simulink model "sm_abbYuMi_trajectory"  (R2021a)
settings: Solver=daessc  StartTime=0.0  StopTime=size(waypointsL, 2) * segment_duration  MaxStep=0.5  RelTol=1e-3  AbsTol=1e-3
values from neighbouring files (symbols this model uses):
  cube_l = 0.02    [startup_sm_abbYuMi_trajectory.m]
  segment_duration = 1.5    [sm_abbYuMi_trajectory_waypoints.m]    (also in startup_sm_abbYuMi_trajectory.m = 2)
undefined symbols (not defined in the file or in its folder): F1, F2, X, Y, Z
libraries: sm_lib x228, nesl_utility x52, robotcorelib x2
(part 1 of 6)
CloseFcn:
  | try,close(h1_sm_abbYuMi_trajectory),end
  | clear h1_sm_abbYuMi_2_trajectory
  | try,close(h2_sm_abbYuMi_trajectory),end
  | clear h2_sm_abbYuMi_2_trajectory
  | try,close(h3_sm_abbYuMi_trajectory),end
  | clear h3_sm_abbYuMi_2_trajectory
  | try,close(h4_sm_abbYuMi_trajectory),end
  | clear h4_sm_abbYuMi_trajectory
  | 
  | 
  | clear simlog_sm_abbYuMi_trajectory
  | clear logsout_sm_abbYuMi_trajectory
Description:
  | Dual Arm Robot Trajectory Testing
settings Model: Creator=smiller  LastModifiedBy=USER
settings SolverCC: AutoScaleAbsTol=off
settings DataIOCC: MaxDataPoints=10000  ReturnWorkspaceOutputs=off  SignalLoggingName=logsout_sm_abbYuMi_trajectory
settings SimscapeCC: SimscapeLogType=all  SimscapeLogSimulationStatistics=on  SimscapeLogName=simlog_sm_abbYuMi_trajectory  SimscapeLogDataHistory=10000
settings ExplorerConfigSet: InternalSimMechanicsExplorerSettings="<ExplorerConfiguration><canonicalview>default</canonicalview><AnimationSetting><BasePlaybackSpeed>1.0</BasePlaybackSpeed><PlaybackSpeedFactor>1.0</PlaybackSpeedFactor></AnimationSetting><TilePanel><TileInfo><Tiles Columns=\"1\" Count=\"1\" Rows=\"1\"><Column Weight=\"1\"/><Row Weight=\"1\"/><Tile Height=\"1\" Width=\"1\" X=\"0\" Y=\"0\"/></Tiles></TileInfo><SceneInfo><SceneViewer><BGColor><R>1</R><G>1</G><B>1</B></BGColor><Camera><DoPerspective>off</DoPerspective><Position><X>0.471611663595321084</X><Y>-0.677761083071622084</Y><Z>0.849724510093532892</Z></Position><Center><X>-0.196535950699227191</X><Y>-0.00961346877707375258</Y><Z>0.181576895798984672</Z></Center><Up><X>-0.408248290463863073</X><Y>0.408248290463863073</Y><Z>0.816496580927726145</Z></Up><ViewLimDist>1</ViewLimDist><YLim>0.557252171635627791</YLim><XLim>0.800218953628602181</XLim></Camera></SceneViewer></SceneInfo></TilePanel><MechEditorPanel><Cameras/><GfxPanelCameraMap/><VideoCreator><PlaybackSpeedRatio>1</PlaybackSpeedRatio><FrameRate>30</FrameRate><VideoFormat>MPEG-4</VideoFormat><FrameSize>auto</FrameSize></VideoCreator></MechEditorPanel></ExplorerConfiguration>"

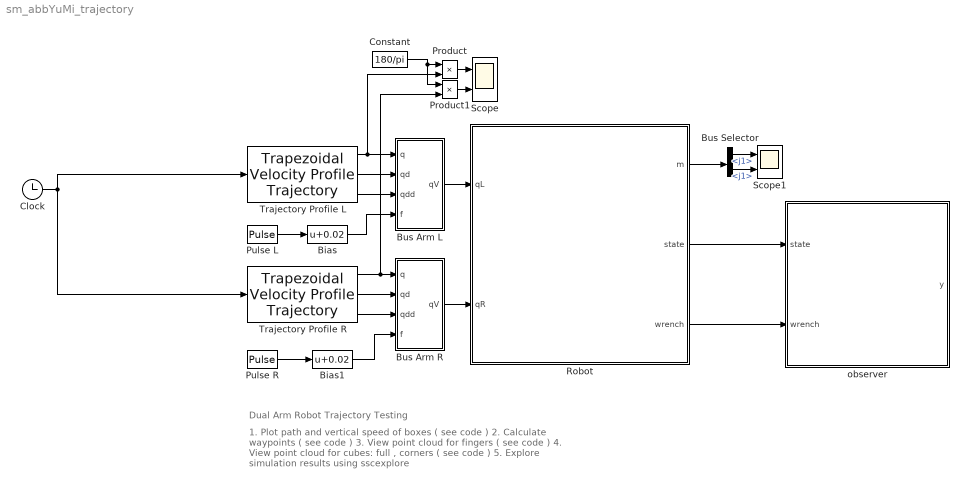
== system sm_abbYuMi_trajectory ==
  note: Dual Arm Robot Trajectory Testing
  note: 1. Plot path and vertical speed of boxes ( see code )
      | 2. Calculate waypoints ( see code )
      | 3. View point cloud for fingers ( see code )
      | 4. View point cloud for cubes: full , corners ( see code )
      | 5. Explore simulation results using sscexplore
  Bias : Bias  Bias=0.02
  Bias1 : Bias  Bias=0.02
  Bus Selector : BusSelector  OutputSignals=trqL.j1,trqR.j1
  Bus Arm L : Subsystem
  Bus Arm R : Subsystem
  Clock : Clock
  Constant : Constant  Value=180/pi
  Product : Product
  Product1 : Product
  Pulse L : DiscretePulseGenerator  PulseType=Time based  Amplitude=-0.011  Period=100  PulseWidth=4*segment_duration  PhaseDelay=2*segment_duration
  Pulse R : DiscretePulseGenerator  PulseType=Time based  Amplitude=-0.011  Period=100  PulseWidth=4*segment_duration  PhaseDelay=6*segment_duration
  Robot : Subsystem  mask(Dual Arm Robot with Contact Forces){k_gripBox=1e3, k_boxBox=1e3, k_boxFloor=1e3, d_gripBox=1e2, d_boxBox=1e2, d_boxFloor=1e2, t_gripBox=1e-3, t_boxBox=1e-3, t_boxFloor=1e-3, mu_s_gripBox=0.7, mu_s_boxBox=0.5, mu_s_boxFloor=0.5, mu_d_gripBox=0.5, mu_d_boxBox=0.3, mu_d_boxFloor=0.3, mu_v_gripBox=1e-3, mu_v_boxBox=1e-3, mu_v_boxFloor=1e-3}
      mask help: Models a dual-arm robot. Parameter values define the contact and friction forces between the gripper, boxes, and floor.
      mask DialogControl Control2_copy_copy_copy_copy_copy_copy_copy Prompt: Gripper-Box
      mask DialogControl Control2_copy_copy_copy_copy_copy_copy_copy_copy Prompt: Box-Box
      mask DialogControl Control2_copy_copy_copy_copy_copy_copy_copy_copy_copy Prompt: Box-Floor
      mask DialogControl Control2_copy_copy_copy_copy_copy_copy Prompt: Damping (N/(m/s))
      mask DialogControl Control2_copy Prompt: Damping (N/(m/s))
      mask DialogControl Control2_copy_copy Prompt: Transition Width (m)
      mask DialogControl Control2_copy_copy_copy Prompt: Static Friction (0-1)
      mask DialogControl Control2_copy_copy_copy_copy Prompt: Dynamic Friction (0-1)
      mask DialogControl Control2_copy_copy_copy_copy_copy Prompt: Critical Velocity (m/s)
      mask Display: image('sm_abbYuMi_trajectory_robot.png');
  Scope : Scope  NumInputPorts=2
  Scope1 : Scope  NumInputPorts=2
  Trajectory Profile L : robotcorelib/Trapezoidal Velocity Profile Trajectory  WaypointSource=Internal  Waypoints=waypointsL  NumParams=1  Parameter1=End Time  Parameter2=End Time  ParameterSource=Internal  PeakVelocity=[ 2; 2 ]  Acceleration=[ 1; 2 ]  EndTime=segment_duration  AccelTime=[ 1; 2 ]  SimulateUsing=Code generation
      settings: SourceProductBaseCode=NV,RO,RR,UV
  Trajectory Profile R : robotcorelib/Trapezoidal Velocity Profile Trajectory  WaypointSource=Internal  Waypoints=waypointsR  NumParams=1  Parameter1=End Time  Parameter2=End Time  ParameterSource=Internal  PeakVelocity=[ 2; 2 ]  Acceleration=[ 1; 2 ]  EndTime=segment_duration  AccelTime=[ 1; 2 ]  SimulateUsing=Code generation
      settings: SourceProductBaseCode=NV,RO,RR,UV
  observer : Subsystem
  wires:
  Clock/1 -> Trajectory Profile L/1, Trajectory Profile R/1
  Trajectory Profile L/1 -> Product/2, Bus Arm L/1(q)
  Trajectory Profile L/2 -> Bus Arm L/2(qd)
  Trajectory Profile L/3 -> Bus Arm L/3(qdd)
  Product/1 -> Scope/1
  Pulse L/1 -> Bias/1
  Trajectory Profile R/3 -> Bus Arm R/3(qdd)
  Trajectory Profile R/2 -> Bus Arm R/2(qd)
  Trajectory Profile R/1 -> Product1/2, Bus Arm R/1(q)
  Product1/1 -> Scope/2
  Pulse R/1 -> Bias1/1
  Bus Arm L/1(qV) -> Robot/1(qL)
  Constant/1 -> Product1/1, Product/1
  Bias1/1 -> Bus Arm R/4(f)
  Bias/1 -> Bus Arm L/4(f)
  Robot/1(m) -> Bus Selector/1
  Bus Selector/1 -> Scope1/1  "<j1>"
  Bus Selector/2 -> Scope1/2  "<j1>"
  Robot/2(state) -> observer/1(state)
  Robot/3(wrench) -> observer/2(wrench)
  Bus Arm R/1(qV) -> Robot/2(qR)

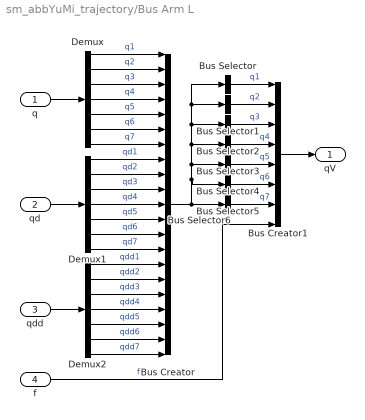
== system sm_abbYuMi_trajectory/Bus Arm L ==
  q : Inport
  qd : Inport  Port=2
  qdd : Inport  Port=3
  f : Inport  Port=4
  Bus Creator : BusCreator  Inputs=21
  Bus Creator1 : BusCreator  Inputs=8
  Bus Selector : BusSelector  OutputSignals=q1,qd1,qdd1  OutputAsBus=on
  Bus Selector1 : BusSelector  OutputSignals=q2,qd2,qdd2  OutputAsBus=on
  Bus Selector2 : BusSelector  OutputSignals=q3,qd3,qdd3  OutputAsBus=on
  Bus Selector3 : BusSelector  OutputSignals=q4,qd4,qdd4  OutputAsBus=on
  Bus Selector4 : BusSelector  OutputSignals=q5,qd5,qdd5  OutputAsBus=on
  Bus Selector5 : BusSelector  OutputSignals=q6,qd6,qdd6  OutputAsBus=on
  Bus Selector6 : BusSelector  OutputSignals=q7,qd7,qdd7  OutputAsBus=on
  Demux : Demux  Outputs=7
  Demux1 : Demux  Outputs=7
  Demux2 : Demux  Outputs=7
  qV : Outport
  wires:
  f/1 -> Bus Creator1/8  "f"
  q/1 -> Demux/1
  qd/1 -> Demux1/1
  qdd/1 -> Demux2/1
  Demux/1 -> Bus Creator/1  "q1"
  Demux/2 -> Bus Creator/2  "q2"
  Demux/3 -> Bus Creator/3  "q3"
  Demux/4 -> Bus Creator/4  "q4"
  Demux/5 -> Bus Creator/5  "q5"
  Demux/6 -> Bus Creator/6  "q6"
  Demux/7 -> Bus Creator/7  "q7"
  Demux1/1 -> Bus Creator/8  "qd1"
  Demux1/2 -> Bus Creator/9  "qd2"
  Demux1/3 -> Bus Creator/10  "qd3"
  Demux1/4 -> Bus Creator/11  "qd4"
  Demux1/5 -> Bus Creator/12  "qd5"
  Demux1/6 -> Bus Creator/13  "qd6"
  Demux1/7 -> Bus Creator/14  "qd7"
  Demux2/1 -> Bus Creator/15  "qdd1"
  Demux2/2 -> Bus Creator/16  "qdd2"
  Demux2/3 -> Bus Creator/17  "qdd3"
  Demux2/4 -> Bus Creator/18  "qdd4"
  Demux2/5 -> Bus Creator/19  "qdd5"
  Demux2/6 -> Bus Creator/20  "qdd6"
  Demux2/7 -> Bus Creator/21  "qdd7"
  Bus Creator/1 -> Bus Selector5/1, Bus Selector4/1, Bus Selector3/1, Bus Selector2/1, Bus Selector/1, Bus Selector1/1, Bus Selector6/1
  Bus Selector/1 -> Bus Creator1/1  "q1"
  Bus Selector1/1 -> Bus Creator1/2  "q2"
  Bus Selector2/1 -> Bus Creator1/3  "q3"
  Bus Selector3/1 -> Bus Creator1/4  "q4"
  Bus Selector4/1 -> Bus Creator1/5  "q5"
  Bus Selector5/1 -> Bus Creator1/6  "q6"
  Bus Selector6/1 -> Bus Creator1/7  "q7"
  Bus Creator1/1 -> qV/1

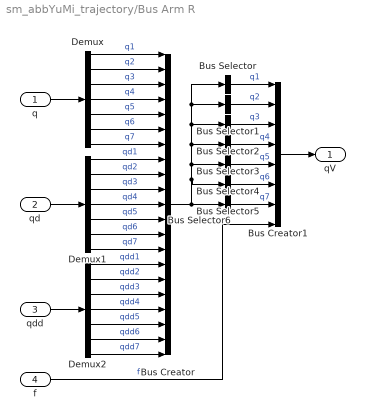
== system sm_abbYuMi_trajectory/Bus Arm R ==
  q : Inport
  qd : Inport  Port=2
  qdd : Inport  Port=3
  f : Inport  Port=4
  Bus Creator : BusCreator  Inputs=21
  Bus Creator1 : BusCreator  Inputs=8
  Bus Selector : BusSelector  OutputSignals=q1,qd1,qdd1  OutputAsBus=on
  Bus Selector1 : BusSelector  OutputSignals=q2,qd2,qdd2  OutputAsBus=on
  Bus Selector2 : BusSelector  OutputSignals=q3,qd3,qdd3  OutputAsBus=on
  Bus Selector3 : BusSelector  OutputSignals=q4,qd4,qdd4  OutputAsBus=on
  Bus Selector4 : BusSelector  OutputSignals=q5,qd5,qdd5  OutputAsBus=on
  Bus Selector5 : BusSelector  OutputSignals=q6,qd6,qdd6  OutputAsBus=on
  Bus Selector6 : BusSelector  OutputSignals=q7,qd7,qdd7  OutputAsBus=on
  Demux : Demux  Outputs=7
  Demux1 : Demux  Outputs=7
  Demux2 : Demux  Outputs=7
  qV : Outport
  wires:
  Bus Creator1/1 -> qV/1
  Bus Selector6/1 -> Bus Creator1/7  "q7"
  Bus Selector5/1 -> Bus Creator1/6  "q6"
  Bus Selector4/1 -> Bus Creator1/5  "q5"
  Bus Selector3/1 -> Bus Creator1/4  "q4"
  Bus Selector2/1 -> Bus Creator1/3  "q3"
  Bus Selector1/1 -> Bus Creator1/2  "q2"
  Bus Selector/1 -> Bus Creator1/1  "q1"
  Bus Creator/1 -> Bus Selector6/1, Bus Selector1/1, Bus Selector/1, Bus Selector2/1, Bus Selector3/1, Bus Selector4/1, Bus Selector5/1
  Demux2/7 -> Bus Creator/21  "qdd7"
  Demux2/6 -> Bus Creator/20  "qdd6"
  Demux2/5 -> Bus Creator/19  "qdd5"
  Demux2/4 -> Bus Creator/18  "qdd4"
  Demux2/3 -> Bus Creator/17  "qdd3"
  Demux2/2 -> Bus Creator/16  "qdd2"
  Demux2/1 -> Bus Creator/15  "qdd1"
  Demux1/7 -> Bus Creator/14  "qd7"
  Demux1/6 -> Bus Creator/13  "qd6"
  Demux1/5 -> Bus Creator/12  "qd5"
  Demux1/4 -> Bus Creator/11  "qd4"
  Demux1/3 -> Bus Creator/10  "qd3"
  Demux1/2 -> Bus Creator/9  "qd2"
  Demux1/1 -> Bus Creator/8  "qd1"
  Demux/7 -> Bus Creator/7  "q7"
  Demux/6 -> Bus Creator/6  "q6"
  Demux/5 -> Bus Creator/5  "q5"
  Demux/4 -> Bus Creator/4  "q4"
  Demux/3 -> Bus Creator/3  "q3"
  Demux/2 -> Bus Creator/2  "q2"
  Demux/1 -> Bus Creator/1  "q1"
  qdd/1 -> Demux2/1
  qd/1 -> Demux1/1
  q/1 -> Demux/1
  f/1 -> Bus Creator1/8  "f"

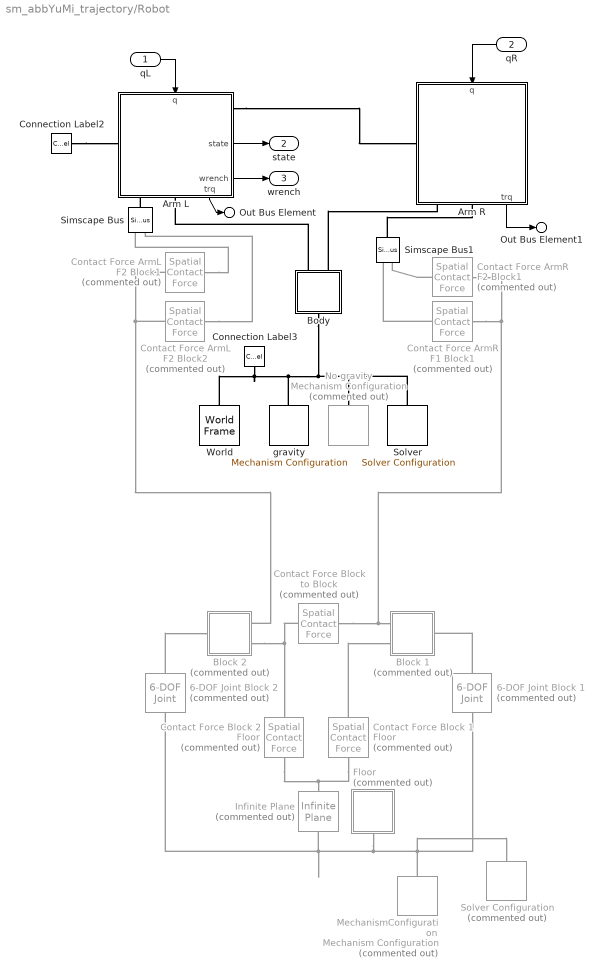
== system sm_abbYuMi_trajectory/Robot ==
  qL : Inport
  qR : Inport  Port=2
  " Contact Force Block to Block" : sm_lib/Forces and Torques/Spatial Contact Force  Commented=on  CoefficientOfDynamicFriction=mu_d_boxBox  CoefficientOfStaticFriction=mu_s_boxBox  SenseContactBaseRotation=off  SenseContactBaseTranslation=off  NormalDamping=d_boxBox  NormalDampingUnits=N/(m/s)  SenseContactFollowerRotation=off  SenseContactFollowerTranslation=off  SenseContactSignal=off  NormalStiffness=k_boxBox  NormalStiffnessUnits=N/m  FrictionalCriticalVelocity=mu_v_boxBox  FrictionalCriticalVelocityUnits=m/s  ZeroCrossDetectContactStartAndEnd=off  FrictionType=SmoothStickSlip  SenseFrictionalForceMagnitude=off  SenseNormalForceMagnitude=off  NormalForceType=SmoothSpringDamper  SenseNormalVelocity=off  SenseSeparationDistance=off  SenseTangentialVelocity=off  SenseTangentialVelocityMagnitude=off  NormalTransitionRegionWidth=t_boxBox  NormalTransitionRegionWidthUnits=m
  6-DOF Joint Block 1 : sm_lib/Joints/6-DOF Joint  Commented=on  JointMode=Normal  SenseConstraintForce=off  SenseConstraintForceX=off  SenseConstraintForceY=off  SenseConstraintForceZ=off  SenseConstraintTorque=off  SenseConstraintTorqueX=off  SenseConstraintTorqueY=off  SenseConstraintTorqueZ=off  SenseTotalForce=off  SenseTotalForceX=off  SenseTotalForceY=off  SenseTotalForceZ=off  SenseTotalTorque=off  SenseTotalTorqueX=off  SenseTotalTorqueY=off  SenseTotalTorqueZ=off  CompositeWrenchDir=FollowerOnBase  CompositeWrenchFrame=BaseFrame  PxEquilibriumPosition=0  PxEquilibriumPositionUnits=m  PxSpringStiffness=0  PxSpringStiffnessUnits=N/m  PxDampingCoefficient=0  PxDampingCoefficientUnits=N/(m/s)  PxTorqueActuationMode=NoTorque  PxMotionActuationMode=ComputedMotion  PxSensePosition=off  PxSenseVelocity=off  PxSenseAcceleration=off  PxSenseTorqueForce=off  PxSenseLowerLimitTorqueForce=off  PxSenseUpperLimitTorqueForce=off  PxLowerLimitSpecify=off  PxLowerLimitBound=-1  PxLowerLimitBoundUnits=m  PxLowerLimitStiffness=1e6  PxLowerLimitStiffnessUnits=N/m  PxLowerLimitDamping=1e3  PxLowerLimitDampingUnits=N/(m/s)  PxLowerLimitTransitionRegionWidth=1e-4  PxLowerLimitTransitionRegionWidthUnits=m  PxUpperLimitSpecify=off  PxUpperLimitBound=1  PxUpperLimitBoundUnits=m  PxUpperLimitStiffness=1e6  PxUpperLimitStiffnessUnits=N/m  PxUpperLimitDamping=1e3  PxUpperLimitDampingUnits=N/(m/s)  PxUpperLimitTransitionRegionWidth=1e-4  PxUpperLimitTransitionRegionWidthUnits=m  PxPositionTargetSpecify=on  PxPositionTargetPriority=High  PxPositionTargetValue=0.1  PxPositionTargetValueUnits=m  PxVelocityTargetSpecify=off  PxVelocityTargetPriority=High  PxVelocityTargetValue=0  PxVelocityTargetValueUnits=m/s  PyEquilibriumPosition=0  PyEquilibriumPositionUnits=m  PySpringStiffness=0  PySpringStiffnessUnits=N/m  PyDampingCoefficient=0  PyDampingCoefficientUnits=N/(m/s)  PyTorqueActuationMode=NoTorque  PyMotionActuationMode=ComputedMotion  PySensePosition=off  PySenseVelocity=off  PySenseAcceleration=off  PySenseTorqueForce=off  PySenseLowerLimitTorqueForce=off  PySenseUpperLimitTorqueForce=off  PyLowerLimitSpecify=off  PyLowerLimitBound=-1  PyLowerLimitBoundUnits=m  PyLowerLimitStiffness=1e6  PyLowerLimitStiffnessUnits=N/m  PyLowerLimitDamping=1e3  PyLowerLimitDampingUnits=N/(m/s)  PyLowerLimitTransitionRegionWidth=1e-4  PyLowerLimitTransitionRegionWidthUnits=m  PyUpperLimitSpecify=off  PyUpperLimitBound=1  PyUpperLimitBoundUnits=m  PyUpperLimitStiffness=1e6  PyUpperLimitStiffnessUnits=N/m  PyUpperLimitDamping=1e3  PyUpperLimitDampingUnits=N/(m/s)  PyUpperLimitTransitionRegionWidth=1e-4  PyUpperLimitTransitionRegionWidthUnits=m  PyPositionTargetSpecify=on  PyPositionTargetPriority=High  PyPositionTargetValue=-0.3  PyPositionTargetValueUnits=m  PyVelocityTargetSpecify=off  PyVelocityTargetPriority=High  PyVelocityTargetValue=0  PyVelocityTargetValueUnits=m/s  PzEquilibriumPosition=0  PzEquilibriumPositionUnits=m  PzSpringStiffness=0  PzSpringStiffnessUnits=N/m  PzDampingCoefficient=0  PzDampingCoefficientUnits=N/(m/s)  PzTorqueActuationMode=NoTorque  PzMotionActuationMode=ComputedMotion  PzSensePosition=off  PzSenseVelocity=off  PzSenseAcceleration=off  PzSenseTorqueForce=off  PzSenseLowerLimitTorqueForce=off  PzSenseUpperLimitTorqueForce=off  PzLowerLimitSpecify=off  PzLowerLimitBound=0  PzLowerLimitBoundUnits=m  PzLowerLimitStiffness=1e6  PzLowerLimitStiffnessUnits=N/m  PzLowerLimitDamping=1e3  PzLowerLimitDampingUnits=N/(m/s)  PzLowerLimitTransitionRegionWidth=1e-4  PzLowerLimitTransitionRegionWidthUnits=m  PzUpperLimitSpecify=off  PzUpperLimitBound=1  PzUpperLimitBoundUnits=m  PzUpperLimitStiffness=1e6  PzUpperLimitStiffnessUnits=N/m  PzUpperLimitDamping=1e3  PzUpperLimitDampingUnits=N/(m/s)  PzUpperLimitTransitionRegionWidth=1e-4  PzUpperLimitTransitionRegionWidthUnits=m  PzPositionTargetSpecify=on  PzPositionTargetPriority=High  PzPositionTargetValue=0.011  PzPositionTargetValueUnits=m  PzVelocityTargetSpecify=off  PzVelocityTargetPriority=High  PzVelocityTargetValue=0  PzVelocityTargetValueUnits=m/s  SphDefPosRotationMethod=None  SphDefPosRotationAngleUnits=deg  SphDefPosRotationStandardAxis=+Z  SphDefPosRotationAngle=0.0  SphDefPosRotationArbitraryAxis=[0 0 1]  SphDefPosFollAlignAxisA=+X  SphDefPosBaseAlignAxisA=+Y  SphDefPosFollAlignAxisB=+Y  SphDefPosBaseAlignAxisB=+Z  SphDefPosRotationSequenceAxes=FollowerAxes  SphDefPosRotationSequence=XYX  SphDefPosRotationSequenceAngles=[0 0 0]  SphDefPosRotationSequenceAnglesUnits=deg  SphDefPosRotationMatrix=[1 0 0; 0 1 0; 0 0 1]  SphEqPosRotationMethod=None  SphEqPosRotationAngleUnits=deg  SphEqPosRotationStandardAxis=+Z  SphEqPosRotationAngle=0.0  SphEqPosRotationArbitraryAxis=[0 0 1]  SphEqPosFollAlignAxisA=+X  SphEqPosBaseAlignAxisA=+Y  SphEqPosFollAlignAxisB=+Y  SphEqPosBaseAlignAxisB=+Z  SphEqPosRotationSequenceAxes=FollowerAxes  SphEqPosRotationSequence=XYX  SphEqPosRotationSequenceAngles=[0 0 0]  SphEqPosRotationSequenceAnglesUnits=deg  SphEqPosRotationMatrix=[1 0 0; 0 1 0; 0 0 1]  SphSpringStiffness=0  SphSpringStiffnessUnits=N*m/deg  SphDampingCoefficient=0  SphDampingCoefficientUnits=N*m/(deg/s)  SphActuateTorqueX=off  SphActuateTorqueY=off  SphActuateTorqueZ=off  SphActuateTorque=off  SphTorqueActuationMode=NoTorque  SphMotionActuationMode=ComputedMotion  SphActuationFrame=BaseFrame  SphSensePosition=off  SphSenseVelocityX=off  SphSenseVelocityY=off  SphSenseVelocityZ=off  SphSenseVelocity=off  SphSenseAccelerationX=off  SphSenseAccelerationY=off  SphSenseAccelerationZ=off  SphSenseAcceleration=off  SphSenseTorqueX=off  SphSenseTorqueY=off  SphSenseTorqueZ=off  SphSenseTorqueForce=off  SphSenseLowerLimitTorqueMag=off  SphSenseUpperLimitTorqueMag=off  SphSensingFrame=BaseFrame  SphLowerLimitSpecify=off  SphLowerLimitBound=15  SphLowerLimitBoundUnits=deg  SphLowerLimitStiffness=1e4  SphLowerLimitStiffnessUnits=N*m/deg  SphLowerLimitDamping=10  SphLowerLimitDampingUnits=N*m/(deg/s)  SphLowerLimitTransitionRegionWidth=0.1  SphLowerLimitTransitionRegionWidthUnits=deg  SphUpperLimitSpecify=off  SphUpperLimitBound=45  SphUpperLimitBoundUnits=deg  SphUpperLimitStiffness=1e4  SphUpperLimitStiffnessUnits=N*m/deg  SphUpperLimitDamping=10  SphUpperLimitDampingUnits=N*m/(deg/s)  SphUpperLimitTransitionRegionWidth=0.1  SphUpperLimitTransitionRegionWidthUnits=deg  SphPositionTargetRotationMethod=None  SphPositionTargetRotationAngleUnits=deg  SphPositionTargetRotationStandardAxis=+Z  SphPositionTargetRotationAngle=0.0  SphPositionTargetRotationArbitraryAxis=[0 0 1]  SphPositionTargetFollAlignAxisA=+X  SphPositionTargetBaseAlignAxisA=+Y  SphPositionTargetFollAlignAxisB=+Y  SphPositionTargetBaseAlignAxisB=+Z  SphPositionTargetRotationSequenceAxes=FollowerAxes  SphPositionTargetRotationSequence=XYX  SphPositionTargetRotationSequenceAngles=[0 0 0]  SphPositionTargetRotationSequenceAnglesUnits=deg  SphPositionTargetRotationMatrix=[1 0 0; 0 1 0; 0 0 1]  SphPositionTargetSpecify=off  SphPositionTargetPriority=High  SphVelocityTargetValue=[0 0 0]  SphVelocityTargetValueUnits=deg/s  SphVelocityTargetSpecify=off  SphVelocityTargetPriority=High  SphVelocityTargetInFollowerFrame=on
  6-DOF Joint Block 2 : sm_lib/Joints/6-DOF Joint  Commented=on  JointMode=Normal  SenseConstraintForce=off  SenseConstraintForceX=off  SenseConstraintForceY=off  SenseConstraintForceZ=off  SenseConstraintTorque=off  SenseConstraintTorqueX=off  SenseConstraintTorqueY=off  SenseConstraintTorqueZ=off  SenseTotalForce=off  SenseTotalForceX=off  SenseTotalForceY=off  SenseTotalForceZ=off  SenseTotalTorque=off  SenseTotalTorqueX=off  SenseTotalTorqueY=off  SenseTotalTorqueZ=off  CompositeWrenchDir=FollowerOnBase  CompositeWrenchFrame=BaseFrame  PxEquilibriumPosition=0  PxEquilibriumPositionUnits=m  PxSpringStiffness=0  PxSpringStiffnessUnits=N/m  PxDampingCoefficient=0  PxDampingCoefficientUnits=N/(m/s)  PxTorqueActuationMode=NoTorque  PxMotionActuationMode=ComputedMotion  PxSensePosition=off  PxSenseVelocity=off  PxSenseAcceleration=off  PxSenseTorqueForce=off  PxSenseLowerLimitTorqueForce=off  PxSenseUpperLimitTorqueForce=off  PxLowerLimitSpecify=off  PxLowerLimitBound=-1  PxLowerLimitBoundUnits=m  PxLowerLimitStiffness=1e6  PxLowerLimitStiffnessUnits=N/m  PxLowerLimitDamping=1e3  PxLowerLimitDampingUnits=N/(m/s)  PxLowerLimitTransitionRegionWidth=1e-4  PxLowerLimitTransitionRegionWidthUnits=m  PxUpperLimitSpecify=off  PxUpperLimitBound=1  PxUpperLimitBoundUnits=m  PxUpperLimitStiffness=1e6  PxUpperLimitStiffnessUnits=N/m  PxUpperLimitDamping=1e3  PxUpperLimitDampingUnits=N/(m/s)  PxUpperLimitTransitionRegionWidth=1e-4  PxUpperLimitTransitionRegionWidthUnits=m  PxPositionTargetSpecify=on  PxPositionTargetPriority=High  PxPositionTargetValue=0.1  PxPositionTargetValueUnits=m  PxVelocityTargetSpecify=off  PxVelocityTargetPriority=High  PxVelocityTargetValue=0  PxVelocityTargetValueUnits=m/s  PyEquilibriumPosition=0  PyEquilibriumPositionUnits=m  PySpringStiffness=0  PySpringStiffnessUnits=N/m  PyDampingCoefficient=0  PyDampingCoefficientUnits=N/(m/s)  PyTorqueActuationMode=NoTorque  PyMotionActuationMode=ComputedMotion  PySensePosition=off  PySenseVelocity=off  PySenseAcceleration=off  PySenseTorqueForce=off  PySenseLowerLimitTorqueForce=off  PySenseUpperLimitTorqueForce=off  PyLowerLimitSpecify=off  PyLowerLimitBound=-1  PyLowerLimitBoundUnits=m  PyLowerLimitStiffness=1e6  PyLowerLimitStiffnessUnits=N/m  PyLowerLimitDamping=1e3  PyLowerLimitDampingUnits=N/(m/s)  PyLowerLimitTransitionRegionWidth=1e-4  PyLowerLimitTransitionRegionWidthUnits=m  PyUpperLimitSpecify=off  PyUpperLimitBound=1  PyUpperLimitBoundUnits=m  PyUpperLimitStiffness=1e6  PyUpperLimitStiffnessUnits=N/m  PyUpperLimitDamping=1e3  PyUpperLimitDampingUnits=N/(m/s)  PyUpperLimitTransitionRegionWidth=1e-4  PyUpperLimitTransitionRegionWidthUnits=m  PyPositionTargetSpecify=on  PyPositionTargetPriority=High  PyPositionTargetValue=0.3  PyPositionTargetValueUnits=m  PyVelocityTargetSpecify=off  PyVelocityTargetPriority=High  PyVelocityTargetValue=0  PyVelocityTargetValueUnits=m/s  PzEquilibriumPosition=0  PzEquilibriumPositionUnits=m  PzSpringStiffness=0  PzSpringStiffnessUnits=N/m  PzDampingCoefficient=0  PzDampingCoefficientUnits=N/(m/s)  PzTorqueActuationMode=NoTorque  PzMotionActuationMode=ComputedMotion  PzSensePosition=off  PzSenseVelocity=off  PzSenseAcceleration=off  PzSenseTorqueForce=off  PzSenseLowerLimitTorqueForce=off  PzSenseUpperLimitTorqueForce=off  PzLowerLimitSpecify=off  PzLowerLimitBound=0  PzLowerLimitBoundUnits=m  PzLowerLimitStiffness=1e6  PzLowerLimitStiffnessUnits=N/m  PzLowerLimitDamping=1e3  PzLowerLimitDampingUnits=N/(m/s)  PzLowerLimitTransitionRegionWidth=1e-4  PzLowerLimitTransitionRegionWidthUnits=m  PzUpperLimitSpecify=off  PzUpperLimitBound=1  PzUpperLimitBoundUnits=m  PzUpperLimitStiffness=1e6  PzUpperLimitStiffnessUnits=N/m  PzUpperLimitDamping=1e3  PzUpperLimitDampingUnits=N/(m/s)  PzUpperLimitTransitionRegionWidth=1e-4  PzUpperLimitTransitionRegionWidthUnits=m  PzPositionTargetSpecify=on  PzPositionTargetPriority=High  PzPositionTargetValue=0.011  PzPositionTargetValueUnits=m  PzVelocityTargetSpecify=off  PzVelocityTargetPriority=High  PzVelocityTargetValue=0  PzVelocityTargetValueUnits=m/s  SphDefPosRotationMethod=None  SphDefPosRotationAngleUnits=deg  SphDefPosRotationStandardAxis=+Z  SphDefPosRotationAngle=0.0  SphDefPosRotationArbitraryAxis=[0 0 1]  SphDefPosFollAlignAxisA=+X  SphDefPosBaseAlignAxisA=+Y  SphDefPosFollAlignAxisB=+Y  SphDefPosBaseAlignAxisB=+Z  SphDefPosRotationSequenceAxes=FollowerAxes  SphDefPosRotationSequence=XYX  SphDefPosRotationSequenceAngles=[0 0 0]  SphDefPosRotationSequenceAnglesUnits=deg  SphDefPosRotationMatrix=[1 0 0; 0 1 0; 0 0 1]  SphEqPosRotationMethod=None  SphEqPosRotationAngleUnits=deg  SphEqPosRotationStandardAxis=+Z  SphEqPosRotationAngle=0.0  SphEqPosRotationArbitraryAxis=[0 0 1]  SphEqPosFollAlignAxisA=+X  SphEqPosBaseAlignAxisA=+Y  SphEqPosFollAlignAxisB=+Y  SphEqPosBaseAlignAxisB=+Z  SphEqPosRotationSequenceAxes=FollowerAxes  SphEqPosRotationSequence=XYX  SphEqPosRotationSequenceAngles=[0 0 0]  SphEqPosRotationSequenceAnglesUnits=deg  SphEqPosRotationMatrix=[1 0 0; 0 1 0; 0 0 1]  SphSpringStiffness=0  SphSpringStiffnessUnits=N*m/deg  SphDampingCoefficient=0  SphDampingCoefficientUnits=N*m/(deg/s)  SphActuateTorqueX=off  SphActuateTorqueY=off  SphActuateTorqueZ=off  SphActuateTorque=off  SphTorqueActuationMode=NoTorque  SphMotionActuationMode=ComputedMotion  SphActuationFrame=BaseFrame  SphSensePosition=off  SphSenseVelocityX=off  SphSenseVelocityY=off  SphSenseVelocityZ=off  SphSenseVelocity=off  SphSenseAccelerationX=off  SphSenseAccelerationY=off  SphSenseAccelerationZ=off  SphSenseAcceleration=off  SphSenseTorqueX=off  SphSenseTorqueY=off  SphSenseTorqueZ=off  SphSenseTorqueForce=off  SphSenseLowerLimitTorqueMag=off  SphSenseUpperLimitTorqueMag=off  SphSensingFrame=BaseFrame  SphLowerLimitSpecify=off  SphLowerLimitBound=15  SphLowerLimitBoundUnits=deg  SphLowerLimitStiffness=1e4  SphLowerLimitStiffnessUnits=N*m/deg  SphLowerLimitDamping=10  SphLowerLimitDampingUnits=N*m/(deg/s)  SphLowerLimitTransitionRegionWidth=0.1  SphLowerLimitTransitionRegionWidthUnits=deg  SphUpperLimitSpecify=off  SphUpperLimitBound=45  SphUpperLimitBoundUnits=deg  SphUpperLimitStiffness=1e4  SphUpperLimitStiffnessUnits=N*m/deg  SphUpperLimitDamping=10  SphUpperLimitDampingUnits=N*m/(deg/s)  SphUpperLimitTransitionRegionWidth=0.1  SphUpperLimitTransitionRegionWidthUnits=deg  SphPositionTargetRotationMethod=None  SphPositionTargetRotationAngleUnits=deg  SphPositionTargetRotationStandardAxis=+Z  SphPositionTargetRotationAngle=0.0  SphPositionTargetRotationArbitraryAxis=[0 0 1]  SphPositionTargetFollAlignAxisA=+X  SphPositionTargetBaseAlignAxisA=+Y  SphPositionTargetFollAlignAxisB=+Y  SphPositionTargetBaseAlignAxisB=+Z  SphPositionTargetRotationSequenceAxes=FollowerAxes  SphPositionTargetRotationSequence=XYX  SphPositionTargetRotationSequenceAngles=[0 0 0]  SphPositionTargetRotationSequenceAnglesUnits=deg  SphPositionTargetRotationMatrix=[1 0 0; 0 1 0; 0 0 1]  SphPositionTargetSpecify=off  SphPositionTargetPriority=High  SphVelocityTargetValue=[0 0 0]  SphVelocityTargetValueUnits=deg/s  SphVelocityTargetSpecify=off  SphVelocityTargetPriority=High  SphVelocityTargetInFollowerFrame=on
  Arm L : Subsystem
      settings: PortSchema="{\"entries\":[{\"content\":{\"sides\":[{\"content\":{\"connectorIds\":[\"In1\"]},\"type\":\"ConnectorPlacement.EquallySpacedRectSide\",\"uuid\":\"bd1dcecf-d297-44c9-a9a5-35bbd8af8960\"},{\"content\":{\"connectorIds\":[\"Out1\",\"RConn1\",\"RConn2\"],\"side\":\"RIGHT\"},\"type\":\"ConnectorPlacement.EquallySpacedRectSide\",\"uuid\":\"baf14d35-3a07-4b12-83f0-83ffbc31cdf5\"},{\"content\":{\"connectorIds\":[\"LConn1\",\"Out2\",\"Out3\"],\"side\":\"TOP\"},\"type\":\"ConnectorPlacement.EquallySpacedRectSide\",\"uuid\":\"824d8d51-c42e-4dae-9a8c-2ffaab279e02\"},{\"content\":{\"connectorIds\":[\"RConn3\"],\"side\":\"BOTTOM\"},\"type\":\"ConnectorPlacement.EquallySpacedRectSide\",\"uuid\":\"ad6f5a81-da03-4abe-8c16-f1c9b20f9016\"}]},\"type\":\"ConnectorPlacement.EquallySpacedConnector\",\"uuid\":\"fe86daed-a59d-484b-b331-148b99957df6\"}],\"packageUris\":[\"http://schema.mathworks.com/mf0/Connector/R2020b\"],\"version\":\"1.0\"}"
  Arm R : Subsystem
      settings: PortSchema="{\"entries\":[{\"content\":{\"sides\":[{\"content\":{\"connectorIds\":[\"In1\"]},\"type\":\"ConnectorPlacement.EquallySpacedRectSide\",\"uuid\":\"a5483abb-2b55-4c80-92c1-57afb39286c9\"},{\"content\":{\"connectorIds\":[\"Out1\",\"RConn1\",\"RConn2\"],\"side\":\"RIGHT\"},\"type\":\"ConnectorPlacement.EquallySpacedRectSide\",\"uuid\":\"70e7c0c0-7b67-4471-83d4-ebce2c38e118\"},{\"content\":{\"connectorIds\":[],\"side\":\"TOP\"},\"type\":\"ConnectorPlacement.EquallySpacedRectSide\",\"uuid\":\"5c3252dc-82b7-4f09-980f-704b78bb4b1e\"},{\"content\":{\"connectorIds\":[\"RConn3\"],\"side\":\"BOTTOM\"},\"type\":\"ConnectorPlacement.EquallySpacedRectSide\",\"uuid\":\"dc850cf4-a88e-4fa0-b309-256fbdf4b05e\"}]},\"type\":\"ConnectorPlacement.EquallySpacedConnector\",\"uuid\":\"ac9f6d8b-81cb-4b9f-aec0-3731a82563a6\"}],\"packageUris\":[\"http://schema.mathworks.com/mf0/Connector/R2020b\"],\"version\":\"1.0\"}"
  Block 1 : Subsystem  Commented=on
  Block 2 : Subsystem  Commented=on
  Body : Subsystem
  Connection Label2 : ConnectionLabel  Label=W
  Connection Label3 : ConnectionLabel  Label=W
  Contact Force Block 1 Floor : sm_lib/Forces and Torques/Spatial Contact Force  Commented=on  CoefficientOfDynamicFriction=mu_d_boxFloor  CoefficientOfStaticFriction=mu_s_boxFloor  SenseContactBaseRotation=off  SenseContactBaseTranslation=off  NormalDamping=d_boxFloor  NormalDampingUnits=N/(m/s)  SenseContactFollowerRotation=off  SenseContactFollowerTranslation=off  SenseContactSignal=off  NormalStiffness=k_boxFloor  NormalStiffnessUnits=N/m  FrictionalCriticalVelocity=mu_v_boxFloor  FrictionalCriticalVelocityUnits=m/s  ZeroCrossDetectContactStartAndEnd=off  FrictionType=SmoothStickSlip  SenseFrictionalForceMagnitude=off  SenseNormalForceMagnitude=off  NormalForceType=SmoothSpringDamper  SenseNormalVelocity=off  SenseSeparationDistance=off  SenseTangentialVelocity=off  SenseTangentialVelocityMagnitude=off  NormalTransitionRegionWidth=t_boxFloor  NormalTransitionRegionWidthUnits=m
  Contact Force Block 2 Floor : sm_lib/Forces and Torques/Spatial Contact Force  Commented=on  CoefficientOfDynamicFriction=mu_d_boxFloor  CoefficientOfStaticFriction=mu_s_boxFloor  SenseContactBaseRotation=off  SenseContactBaseTranslation=off  NormalDamping=d_boxFloor  NormalDampingUnits=N/(m/s)  SenseContactFollowerRotation=off  SenseContactFollowerTranslation=off  SenseContactSignal=off  NormalStiffness=k_boxFloor  NormalStiffnessUnits=N/m  FrictionalCriticalVelocity=mu_v_boxFloor  FrictionalCriticalVelocityUnits=m/s  ZeroCrossDetectContactStartAndEnd=off  FrictionType=SmoothStickSlip  SenseFrictionalForceMagnitude=off  SenseNormalForceMagnitude=off  NormalForceType=SmoothSpringDamper  SenseNormalVelocity=off  SenseSeparationDistance=off  SenseTangentialVelocity=off  SenseTangentialVelocityMagnitude=off  NormalTransitionRegionWidth=t_boxFloor  NormalTransitionRegionWidthUnits=m
  Contact Force ArmL F2 Block1 : sm_lib/Forces and Torques/Spatial Contact Force  Commented=on  CoefficientOfDynamicFriction=mu_d_gripBox  CoefficientOfStaticFriction=mu_s_gripBox  SenseContactBaseRotation=off  SenseContactBaseTranslation=off  NormalDamping=d_gripBox  NormalDampingUnits=N/(m/s)  SenseContactFollowerRotation=off  SenseContactFollowerTranslation=off  SenseContactSignal=off  NormalStiffness=k_gripBox  NormalStiffnessUnits=N/m  FrictionalCriticalVelocity=mu_v_gripBox  FrictionalCriticalVelocityUnits=m/s  ZeroCrossDetectContactStartAndEnd=off  FrictionType=SmoothStickSlip  SenseFrictionalForceMagnitude=off  SenseNormalForceMagnitude=off  NormalForceType=SmoothSpringDamper  SenseNormalVelocity=off  SenseSeparationDistance=off  SenseTangentialVelocity=off  SenseTangentialVelocityMagnitude=off  NormalTransitionRegionWidth=t_gripBox  NormalTransitionRegionWidthUnits=m
  Contact Force ArmL F2 Block2 : sm_lib/Forces and Torques/Spatial Contact Force  Commented=on  CoefficientOfDynamicFriction=mu_d_gripBox  CoefficientOfStaticFriction=mu_s_gripBox  SenseContactBaseRotation=off  SenseContactBaseTranslation=off  NormalDamping=d_gripBox  NormalDampingUnits=N/(m/s)  SenseContactFollowerRotation=off  SenseContactFollowerTranslation=off  SenseContactSignal=off  NormalStiffness=k_gripBox  NormalStiffnessUnits=N/m  FrictionalCriticalVelocity=mu_v_gripBox  FrictionalCriticalVelocityUnits=m/s  ZeroCrossDetectContactStartAndEnd=off  FrictionType=SmoothStickSlip  SenseFrictionalForceMagnitude=off  SenseNormalForceMagnitude=off  NormalForceType=SmoothSpringDamper  SenseNormalVelocity=off  SenseSeparationDistance=off  SenseTangentialVelocity=off  SenseTangentialVelocityMagnitude=off  NormalTransitionRegionWidth=t_gripBox  NormalTransitionRegionWidthUnits=m
  Contact Force ArmR F1 Block1 : sm_lib/Forces and Torques/Spatial Contact Force  Commented=on  CoefficientOfDynamicFriction=mu_d_gripBox  CoefficientOfStaticFriction=mu_s_gripBox  SenseContactBaseRotation=off  SenseContactBaseTranslation=off  NormalDamping=d_gripBox  NormalDampingUnits=N/(m/s)  SenseContactFollowerRotation=off  SenseContactFollowerTranslation=off  SenseContactSignal=off  NormalStiffness=k_gripBox  NormalStiffnessUnits=N/m  FrictionalCriticalVelocity=mu_v_gripBox  FrictionalCriticalVelocityUnits=m/s  ZeroCrossDetectContactStartAndEnd=off  FrictionType=SmoothStickSlip  SenseFrictionalForceMagnitude=off  SenseNormalForceMagnitude=off  NormalForceType=SmoothSpringDamper  SenseNormalVelocity=off  SenseSeparationDistance=off  SenseTangentialVelocity=off  SenseTangentialVelocityMagnitude=off  NormalTransitionRegionWidth=t_gripBox  NormalTransitionRegionWidthUnits=m
  Contact Force ArmR F2 Block1 : sm_lib/Forces and Torques/Spatial Contact Force  Commented=on  CoefficientOfDynamicFriction=mu_d_gripBox  CoefficientOfStaticFriction=mu_s_gripBox  SenseContactBaseRotation=off  SenseContactBaseTranslation=off  NormalDamping=d_gripBox  NormalDampingUnits=N/(m/s)  SenseContactFollowerRotation=off  SenseContactFollowerTranslation=off  SenseContactSignal=off  NormalStiffness=k_gripBox  NormalStiffnessUnits=N/m  FrictionalCriticalVelocity=mu_v_gripBox  FrictionalCriticalVelocityUnits=m/s  ZeroCrossDetectContactStartAndEnd=off  FrictionType=SmoothStickSlip  SenseFrictionalForceMagnitude=off  SenseNormalForceMagnitude=off  NormalForceType=SmoothSpringDamper  SenseNormalVelocity=off  SenseSeparationDistance=off  SenseTangentialVelocity=off  SenseTangentialVelocityMagnitude=off  NormalTransitionRegionWidth=t_gripBox  NormalTransitionRegionWidthUnits=m
  Floor : Subsystem  Commented=on
  Infinite Plane : sm_lib/Curves and Surfaces/Infinite Plane  Commented=on  GraphicType=Rectangle  GraphicPlaneWidth=1  GraphicPlaneWidthUnits=m  GraphicPlaneHeight=1  GraphicPlaneHeightUnits=m  GraphicVisPropType=SimpleVisualProperties  GraphicDiffuseColor=[0.5 0.5 0.5]  GraphicOpacity=0.25  GraphicSpecularColor=[0.5 0.5 0.5 1.0]  GraphicAmbientColor=[0.15 0.15 0.15 1.0]  GraphicEmissiveColor=[0.0 0.0 0.0 1.0]  GraphicShininess=75
  MechanismConfiguration : sm_lib/Utilities/Mechanism Configuration  Commented=on  UniformGravity=Constant  GravityVector=[0 0 0]  GravityVectorUnits=m/s^2  GravityUnits=m/s^2  LinearizationDelta=0.001  JointModeTransitionNonlinearIterations=2
  No gravity : sm_lib/Utilities/Mechanism Configuration  Commented=on  UniformGravity=Constant  GravityVector=[0 0 0]  GravityVectorUnits=m/s^2  GravityUnits=m/s^2  LinearizationDelta=0.001  JointModeTransitionNonlinearIterations=2
  Simscape Bus : SimscapeBus  HierarchyStrings=F1;F2
  Simscape Bus1 : SimscapeBus  HierarchyStrings=F1;F2
  Solver : nesl_utility/Solver Configuration  PhysicalDomain=network_engine_domain  SubClassName=solver  LeftPortType=input  RightPortType=generic  Tones=[]  Harmonics=[]  SimulateNoise=off  Profile=off  UseLocalSampling=off  EnableSwitchedLinearOptims=on  FrequencyDomain=off  UseCCode=off  RelTol=0.001  AbsTol=1e-06  MinStep=1e-09  ToWorkspace=off  RevertToSquareIcSolve=off  NumHomotopyIterations=100  PhasorMode=off  PhasorModeNumHarmonics=1  DoDC=off  ResidualTolerance=1e-09  UseLocalSolver=off  LocalSolverChoice=NE_BACKWARD_EULER_ADVANCER  LocalSolverSampleTime=0.001  DoFixedCost=off  MaxNonlinIter=3  MaxModeIter=2  ComputeImpulses=off  ImpulseIterations=2  LinearAlgebra=auto  EquationFormulation=NE_TIME_EF  DelaysMemoryBudget=1024  AutomaticFiltering=on  FilteringTimeConstant=0.001  PartitionStorageMethod=AS_NEEDED  PartitionMemoryBudget=1024  PartitionMethod=ROBUST
      settings: SourceProductBaseCode=PW,SS
  Solver Configuration : nesl_utility/Solver Configuration  Commented=on  PhysicalDomain=network_engine_domain  SubClassName=solver  LeftPortType=input  RightPortType=generic  Tones=[]  Harmonics=[]  SimulateNoise=off  Profile=off  UseLocalSampling=off  EnableSwitchedLinearOptims=on  FrequencyDomain=off  UseCCode=off  RelTol=0.001  AbsTol=1e-06  MinStep=1e-09  ToWorkspace=off  RevertToSquareIcSolve=off  NumHomotopyIterations=100  PhasorMode=off  PhasorModeNumHarmonics=1  DoDC=off  ResidualTolerance=1e-09  UseLocalSolver=off  LocalSolverChoice=NE_BACKWARD_EULER_ADVANCER  LocalSolverSampleTime=0.001  DoFixedCost=off  MaxNonlinIter=3  MaxModeIter=2  ComputeImpulses=off  ImpulseIterations=2  LinearAlgebra=auto  EquationFormulation=NE_TIME_EF  DelaysMemoryBudget=1024  AutomaticFiltering=on  FilteringTimeConstant=0.001  PartitionStorageMethod=AS_NEEDED  PartitionMemoryBudget=1024  PartitionMethod=ROBUST
      settings: SourceProductBaseCode=PW,SS
  World : sm_lib/Frames and Transforms/World Frame
  gravity : sm_lib/Utilities/Mechanism Configuration  UniformGravity=Constant  GravityVector=[0 0 -9.80665]  GravityVectorUnits=m/s^2  GravityUnits=m/s^2  LinearizationDelta=0.001  JointModeTransitionNonlinearIterations=2
  Out Bus Element : Outport  PortName=m  Element=trqL
  Out Bus Element1 : Outport  PortName=m  Element=trqR
  state : Outport  Port=2
  wrench : Outport  Port=3
  wires:
  qR/1 -> Arm R/1(q)
  qL/1 -> Arm L/1(q)
  Arm L/1(trq) -> Out Bus Element/1
  Arm R/1(trq) -> Out Bus Element1/1
  Arm L/3(wrench) -> wrench/1
  Arm L/2(state) -> state/1
  connections:
  6-DOF Joint Block 1/RConn1 -- Block 1/RConn1
  Contact Force ArmL F2 Block1/RConn1 -- Contact Force ArmL F2 Block2/RConn1 -- Block 2/LConn1
  Block 2/LConn2 -- " Contact Force Block to Block"/LConn1 -- Contact Force Block 2 Floor/LConn1
  MechanismConfiguration/RConn1 -- Solver Configuration/RConn1 -- Infinite Plane/LConn1 -- 6-DOF Joint Block 2/LConn1 -- Floor/LConn1 -- 6-DOF Joint Block 1/LConn1
  Contact Force ArmR F2 Block1/LConn1 -- Simscape Bus1/LConn2
  Contact Force ArmL F2 Block1/LConn1 -- Simscape Bus/LConn1
  Contact Force ArmR F2 Block1/RConn1 -- " Contact Force Block to Block"/RConn1 -- Block 1/LConn1 -- Contact Force ArmR F1 Block1/RConn1
  Simscape Bus/RConn1 -- Arm L/RConn2
  Contact Force Block 2 Floor/RConn1 -- Contact Force Block 1 Floor/RConn1 -- Infinite Plane/RConn1
  Contact Force Block 1 Floor/LConn1 -- Block 1/LConn2
  Simscape Bus1/RConn1 -- Arm R/RConn1
  Contact Force ArmR F1 Block1/LConn1 -- Simscape Bus1/LConn1
  6-DOF Joint Block 2/RConn1 -- Block 2/RConn1
  Contact Force ArmL F2 Block2/LConn1 -- Simscape Bus/LConn2
  Body/RConn1 -- Arm L/RConn1
  Body/RConn2 -- Arm R/RConn2
  Connection Label2/LConn1 -- Arm L/RConn3
  Solver/RConn1 -- gravity/RConn1 -- Connection Label3/LConn1 -- World/RConn1 -- Body/LConn1 -- No gravity/RConn1
  Arm L/LConn1 -- Arm R/RConn3

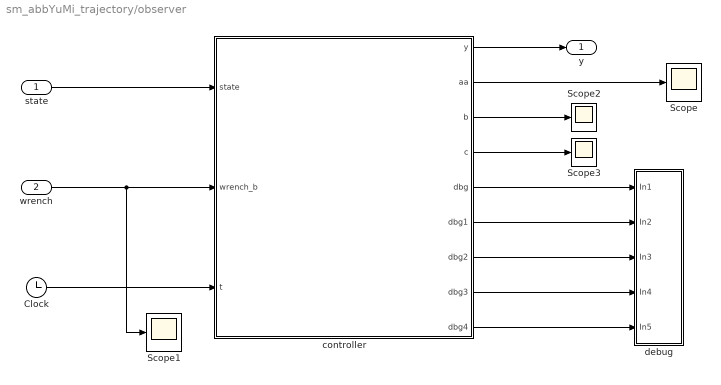
== system sm_abbYuMi_trajectory/observer ==
  state : Inport
  wrench : Inport  Port=2
  Clock : Clock
  Scope{,1..3} (4 alike) : Scope
  controller : MATLAB Function  TreatAsAtomicUnit=on
  debug : Subsystem
  y : Outport
  wires:
  controller/1(y) -> y/1
  state/1 -> controller/1(state)
  controller/5(dbg) -> debug/1(In1)
  controller/2(aa) -> Scope/1
  controller/8(dbg3) -> debug/4(In4)
  controller/6(dbg1) -> debug/2(In2)
  controller/9(dbg4) -> debug/5(In5)
  controller/4(c) -> Scope3/1
  controller/3(b) -> Scope2/1
  controller/7(dbg2) -> debug/3(In3)
  wrench/1 -> Scope1/1, controller/2(wrench_b)
  Clock/1 -> controller/3(t)
